simulink model "quiz2"  (R2022b)
settings: Solver=FixedStepAuto  StartTime=0.0  StopTime=100  FixedStep=0.01  RelTol=1e-3
settings Model: Creator=Fatih  LastModifiedBy=Fatih

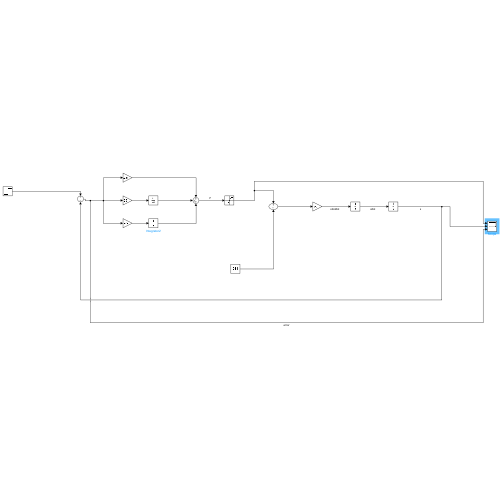
[thumbnail: Simulink's stored preview of the top-level diagram]
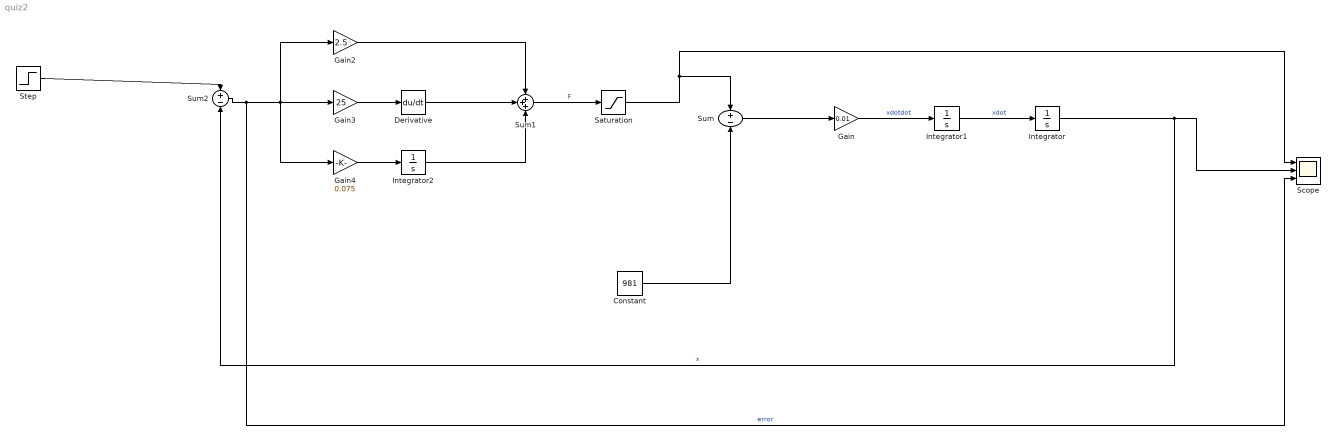
== system quiz2 ==
  Constant : Constant  Value=981
  Derivative : Derivative
  Gain : Gain  Gain=0.01
  Gain2 : Gain  Gain=2.5
  Gain3 : Gain  Gain=25
  Gain4 : Gain  Gain=0.075
  Integrator : Integrator
  Integrator1 : Integrator
  Integrator2 : Integrator
  Saturation : Saturate  UpperLimit=2000
  Scope : Scope  NumInputPorts=3
  Step : Step  Time=0  After=1000  SampleTime=0
  Sum : Sum  Inputs=+-
  Sum1 : Sum  Inputs=+++
  Sum2 : Sum  Inputs=+-
  wires:
  Integrator1/1 -> Integrator/1  "xdot"
  Integrator/1 -> Scope/2, Sum2/2  "x"
  Gain/1 -> Integrator1/1  "xdotdot"
  Sum/1 -> Gain/1
  Sum1/1 -> Saturation/1  "F"
  Gain2/1 -> Sum1/1
  Derivative/1 -> Sum1/2
  Integrator2/1 -> Sum1/3
  Step/1 -> Sum2/1
  Sum2/1 -> Scope/3, Gain2/1, Gain3/1, Gain4/1  "error"
  Gain3/1 -> Derivative/1
  Saturation/1 -> Sum/1, Scope/1
  Constant/1 -> Sum/2
  Gain4/1 -> Integrator2/1
